simulink model "Motor_Cmd_varY_testHarness"  (Simulink 8.0)
settings: Solver=FixedStepDiscrete  StartTime=0.0  StopTime=10  RelTol=1e-3
PreLoadFcn:
  | Motor_Cmd_varY_selfinit
undefined symbols (not defined in the file): sigbuilder_block
settings Model: SldvGeneratedHarnessModel=TestUnitModel=Motor_Cmd_varY|  Creator=fguerin  LastModifiedBy=klindqvi  RecordCoverage=on  CovMetricSettings=dcoe  CovHTMLOptions=-aTS=1 -bRG=1 -bTC=0 -hTR=0 -nFC=0 -scm=1 -bcm=1 -xEv=0  CovCumulativeReport=on  CovReportOnPause=off  CovModelRefEnable=off  CovExternalEMLEnable=on
settings DataIOCC: ExternalInput=SIM_LockDoorRequest  LimitDataPoints=off  SignalLoggingSaveFormat=ModelDataLogs  SaveOutput=off  DSMLogging=off  SaveTime=off  SignalLoggingName=logsOut
settings OptimizationCC: InlineParams=on  InlineInvariantSignals=on  EnhancedBackFolding=on  ZeroExternalMemoryAtStartup=off  ZeroInternalMemoryAtStartup=off  EfficientFloat2IntCast=on  OptimizeModelRefInitCode=on  LifeSpan=1
settings DebuggingCC: SignalInfNanChecking=error  SignalRangeChecking=error  ReadBeforeWriteMsg=EnableAllAsError  WriteAfterWriteMsg=EnableAllAsError  WriteAfterReadMsg=EnableAllAsError  AlgebraicLoopMsg=error  ArtificialAlgebraicLoopMsg=error  SaveWithDisabledLinksMsg=error  SaveWithParameterizedLinksMsg=error  CheckExecutionContextPreStartOutputMsg=on  CheckExecutionContextRuntimeOutputMsg=on  BlockPriorityViolationMsg=error  SolverPrmCheckMsg=error  MultiTaskCondExecSysMsg=warning  MultiTaskRateTransMsg=warning  CheckMatrixSingularityMsg=error  IntegerOverflowMsg=error  ParameterUnderflowMsg=error  ParameterPrecisionLossMsg=error  ParameterTunabilityLossMsg=error  UnderSpecifiedDataTypeMsg=warning  UnnecessaryDatatypeConvMsg=warning  VectorMatrixConversionMsg=error  FcnCallInpInsideContextMsg=EnableAllAsWarning  SFcnCompatibilityMsg=error  BusObjectLabelMismatch=error  RootOutportRequireBusObject=error  AssertControl=DisableAll  ModelReferenceIOMsg=error  ModelReferenceIOMismatchMessage=error  ModelReferenceCSMismatchMessage=warning  UnknownTsInhSupMsg=error  ModelReferenceDataLoggingMessage=error  StrictBusMsg=ErrorOnBusTreatedAsVector
settings HardwareCC: ProdLargestAtomicInteger=Long  ProdLargestAtomicFloat=Double  ProdIntDivRoundTo=Zero  ProdEndianess=BigEndian  ProdHWDeviceType=Freescale->MPC5500
settings ModelReferenceCC: ModelReferenceNumInstancesAllowed=Single
settings SFSimCC: SimParseCustomCode=off
settings RTWCC: SystemTargetFile=ert.tlc  TemplateMakefile=ert_default_tmf  Description=Embedded Coder  GenerateReport=on  RTWVerbose=off  ProcessScript=ert_make_rtw_hook  IncludeHyperlinkInReport=on  LaunchReport=on  PortableWordSizes=on  GenerateTraceInfo=on  GenerateTraceReport=on  GenerateTraceReportSl=on  GenerateTraceReportSf=on  GenerateTraceReportEml=on  GenerateCodeMetricsReport=on
settings MATStruct: className=coder.coverage.Bullseye  argsAllComponents=[]  excludedModels=[]  includeReferencedModels=off  includeTopModel=on  enabled=on
settings CodeAppCC: ForceParamTrailComments=on  IgnoreCustomStorageClasses=off  IgnoreTestpoints=on  MangleLength=4  InlinedPrmAccess=Macros  ReqsInCode=on
settings ERTTargetCC: CodeReplacementLibrary=ANSI_C  MultiwordLength=2048  GenerateSampleERTMain=on  SupportAbsoluteTime=off  SupportNonFinite=off  SupportComplex=off  InlinedParameterPlacement=NonHierarchical  ERTCustomFileTemplate=example_file_process.tlc  ConvertIfToSwitch=off  SuppressUnreachableDefaultCases=off
settings ConfigComp: Description=Design Verifier Custom Configuration Component  DVMaxProcessTime=600  DVDisplayUnsatisfiableObjectives=on  DVAutomaticStubbing=off  DVOutputDir=C:\Work\Data\Pilots\P_PSA_ECoder_BenchMark_LaGarenne\source9b\deliverable\trunk\demos\VnV_example\Projects\ADL_Project/Simulink_Test_Generation/ADL_Sim  DVModelCoverageObjectives=MCDC  DVTestSuiteOptimization=CombinedObjectives  DVDataFileName=./Tests/$ModelName$_sldvdata  DVSaveHarnessModel=on  DVHarnessModelFileName=./Tests/$ModelName$_testHarness  DVModelReferenceHarness=on  DVSaveReport=on  DVReportFileName=ADL_Sim_SLDV.html

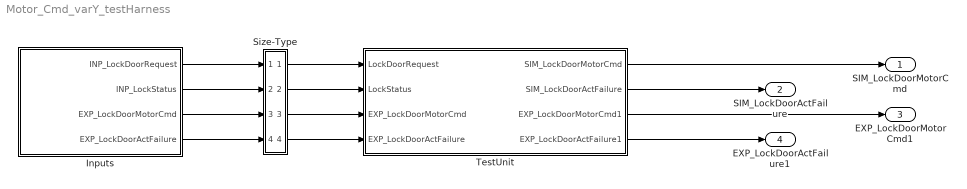
== system Motor_Cmd_varY_testHarness ==
  Inputs : Subsystem  Tag=STV Subsys  RequirementInfo={'other' '..\..\..\..\requirements\doorlockingsystem_swr.doc' '@Simulink_requirement_item_3' 'true' 'REQ301 – A door lock failure should be reported if the door lock has not responded to command in 2 seconds.' '' } %GIDa_ed3108d7_bd27_4d13_a0b7_ca84d234bb27  LoadFcn=sigbuilder_block('load');  StartFcn=sigbuilder_block('start');  StopFcn=sigbuilder_block('stop');  ClipboardFcn=sigbuilder_block('clipboard');  SystemSampleTime=1  mask(Sigbuilder block){}
      mask init:
      | if ~strcmp(get_param(bdroot(gcb),'SimulationStatus'),'stopped'),tuvar = sigbuilder_block('maskInit'); end
      settings: CopyFcn=sigbuilder_block('copy');  DeleteFcn=sigbuilder_block('delete');  ModelCloseFcn=sigbuilder_block('modelClose');  PreSaveFcn=sigbuilder_block('preSave');  PauseFcn=sigbuilder_block('pause')  ContinueFcn=sigbuilder_block('continue')  NameChangeFcn=sigbuilder_block('namechange');  OpenFcn=sigbuilder_block('open',[55.5 107.25 519.75 399.75 ]);  CloseFcn=sigbuilder_block('close');
      mask Display: plot(0, 0, 100, 100,[2, 2, 32, 32, 2], [68, 8, 8, 68, 68],[32, 2], [38, 38], [32, 19, 2],[53, 60, 44], [32, 17, 17, 2],[16, 16, 31, 31]);txt = getActiveGroup(gcbh);text(2, 100, txt,'verticalAlignment', 'top');
  Size-Type : Subsystem
  TestUnit : Subsystem
  SIM_LockDoorMotorCmd : Outport  OutDataTypeStr=uint8  PortDimensions=1
  SIM_LockDoorActFailure : Outport  Port=2  OutDataTypeStr=boolean
  EXP_LockDoorMotorCmd1 : Outport  Port=3  PortDimensions=1
  EXP_LockDoorActFailure1 : Outport  Port=4
  wires:
  Size-Type/1(Out1) -> TestUnit/1(LockDoorRequest)
  Size-Type/2(Out2) -> TestUnit/2(LockStatus)
  Size-Type/3(Out3) -> TestUnit/3(EXP_LockDoorMotorCmd)
  Size-Type/4(Out4) -> TestUnit/4(EXP_LockDoorActFailure)
  TestUnit/1(SIM_LockDoorMotorCmd) -> SIM_LockDoorMotorCmd/1
  TestUnit/2(SIM_LockDoorActFailure) -> SIM_LockDoorActFailure/1
  TestUnit/3(EXP_LockDoorMotorCmd1) -> EXP_LockDoorMotorCmd1/1
  TestUnit/4(EXP_LockDoorActFailure1) -> EXP_LockDoorActFailure1/1
  Inputs/1(INP_LockDoorRequest) -> Size-Type/1(In1)
  Inputs/2(INP_LockStatus) -> Size-Type/2(In2)
  Inputs/3(EXP_LockDoorMotorCmd) -> Size-Type/3(In3)
  Inputs/4(EXP_LockDoorActFailure) -> Size-Type/4(In4)

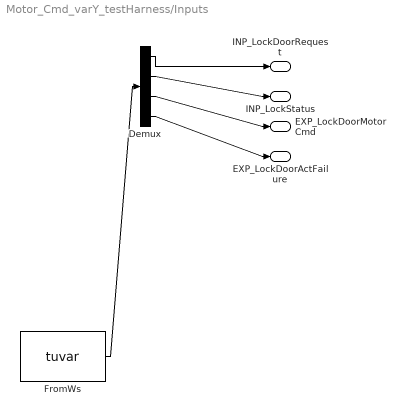
== system Motor_Cmd_varY_testHarness/Inputs ==
  Demux : Demux  Tag=STV Demux
  FromWs : FromWorkspace  Tag=STV FromWs  VariableName=tuvar  SampleTime=0  SigBuilderData=DataTag0  VnvData=DataTag1
      SigBuilderData=|
      | dataSet(1).timeRange = [0 10]
      | dataSet(1).name = 'Test1'
      | dataSet(2).timeRange = [0 10]
      | dataSet(2).name = 'Test2'
      | dataSet(3).timeRange = [0 10]
      | dataSet(3).name = 'Test3'
      | sbobj.Name = 'Signal Builder'
      | sbobj.Groups(1).Name = 'Test1'
      | sbobj.Groups(1).Signals(1).Name = 'INP_LockDoorRequest'
      | sbobj.Groups(1).Signals(1).XData = [0 10]
      | sbobj.Groups(1).Signals(1).YData = [0 0]
      | sbobj.Groups(1).Signals(2).Name = 'INP_LockStatus'
      | sbobj.Groups(1).Signals(2).XData = [0 10]
      | sbobj.Groups(1).Signals(2).YData = [0 0]
      | sbobj.Groups(1).Signals(3).Name = 'EXP_LockDoorMotorCmd'
      | sbobj.Groups(1).Signals(3).XData = [0 10]
      | sbobj.Groups(1).Signals(3).YData = [0 0]
      | sbobj.Groups(1).Signals(4).Name = 'EXP_LockDoorActFailure'
      | sbobj.Groups(1).Signals(4).XData = [0 10]
      | sbobj.Groups(1).Signals(4).YData = [0 0]
      | sbobj.Groups(2).Name = 'Test2'
      | sbobj.Groups(2).Signals(1).Name = 'INP_LockDoorRequest'
      | sbobj.Groups(2).Signals(1).XData = [0 1 1 2 10]
      | sbobj.Groups(2).Signals(1).YData = [0 0 1 1 1]
      | sbobj.Groups(2).Signals(2).Name = 'INP_LockStatus'
      | sbobj.Groups(2).Signals(2).XData = [0 1 1 2 2 10]
      | sbobj.Groups(2).Signals(2).YData = [0 0 0 0 1 1]
      | sbobj.Groups(2).Signals(3).Name = 'EXP_LockDoorMotorCmd'
      | sbobj.Groups(2).Signals(3).XData = [0 1 1 2 2 10]
      | sbobj.Groups(2).Signals(3).YData = [0 0 40 40 40 40]
      | sbobj.Groups(2).Signals(4).Name = 'EXP_LockDoorActFailure'
      | sbobj.Groups(2).Signals(4).XData = [0 1 1 2 2 10]
      | sbobj.Groups(2).Signals(4).YData = [0 0 0 0 0 0]
      | sbobj.Groups(3).Name = 'Test3'
      | sbobj.Groups(3).Signals(1).Name = 'INP_LockDoorRequest'
      | sbobj.Groups(3).Signals(1).XData = [0 1 1 2 10]
      | sbobj.Groups(3).Signals(1).YData = [0 0 1 1 1]
      | sbobj.Groups(3).Signals(2).Name = 'INP_LockStatus'
      | sbobj.Groups(3).Signals(2).XData = [0 1 2 10]
      | sbobj.Groups(3).Signals(2).YData = [0 0 0 0]
      | sbobj.Groups(3).Signals(3).Name = 'EXP_LockDoorMotorCmd'
      | sbobj.Groups(3).Signals(3).XData = [0 1 1 2 10]
      | sbobj.Groups(3).Signals(3).YData = [0 0 40 40 40]
      | sbobj.Groups(3).Signals(4).Name = 'EXP_LockDoorActFailure'
      | sbobj.Groups(3).Signals(4).XData = [0 1 2 3 3 10]
      | sbobj.Groups(3).Signals(4).YData = [0 0 0 0 1 1]
  INP_LockDoorRequest : Outport
  INP_LockStatus : Outport  Tag=STV Outport  Port=2
  EXP_LockDoorMotorCmd : Outport  Tag=STV Outport  Port=3
  EXP_LockDoorActFailure : Outport  Tag=STV Outport  Port=4
  wires:
  FromWs/1 -> Demux/1
  Demux/1 -> INP_LockDoorRequest/1
  Demux/2 -> INP_LockStatus/1
  Demux/3 -> EXP_LockDoorMotorCmd/1
  Demux/4 -> EXP_LockDoorActFailure/1

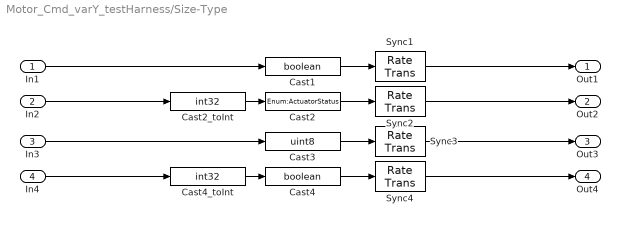
== system Motor_Cmd_varY_testHarness/Size-Type ==
  In1 : Inport
  In2 : Inport  Port=2
  In3 : Inport  Port=3
  In4 : Inport  Port=4
  Cast1 : DataTypeConversion  OutDataTypeStr=boolean  SaturateOnIntegerOverflow=on  RndMeth=Zero
  Cast2 : DataTypeConversion  OutDataTypeStr=Enum:ActuatorStatus  SaturateOnIntegerOverflow=on  RndMeth=Zero
  Cast2_toInt : DataTypeConversion  OutDataTypeStr=int32  SaturateOnIntegerOverflow=on  RndMeth=Zero
  Cast3 : DataTypeConversion  OutDataTypeStr=uint8  SaturateOnIntegerOverflow=on  RndMeth=Zero
  Cast4 : DataTypeConversion  OutDataTypeStr=boolean  SaturateOnIntegerOverflow=on  RndMeth=Zero
  Cast4_toInt : DataTypeConversion  OutDataTypeStr=int32  SaturateOnIntegerOverflow=on  RndMeth=Zero
  Sync{1..4} (4 alike) : RateTransition  OutPortSampleTime=0.5
  Out1 : Outport
  Out2 : Outport  Port=2
  Out3 : Outport  Port=3
  Out4 : Outport  Port=4
  wires:
  In1/1 -> Cast1/1
  Cast1/1 -> Sync1/1
  Sync1/1 -> Out1/1
  In2/1 -> Cast2_toInt/1
  Cast2_toInt/1 -> Cast2/1
  Cast2/1 -> Sync2/1
  Sync2/1 -> Out2/1
  In3/1 -> Cast3/1
  Cast3/1 -> Sync3/1
  Sync3/1 -> Out3/1
  In4/1 -> Cast4_toInt/1
  Cast4_toInt/1 -> Cast4/1
  Cast4/1 -> Sync4/1
  Sync4/1 -> Out4/1

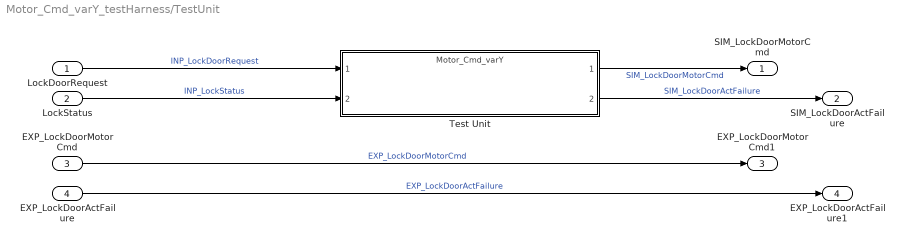
== system Motor_Cmd_varY_testHarness/TestUnit ==
  LockDoorRequest : Inport  OutDataTypeStr=boolean  PortDimensions=1
  LockStatus : Inport  Port=2  OutDataTypeStr=Enum: ActuatorStatus  PortDimensions=1
  EXP_LockDoorMotorCmd : Inport  Port=3  PortDimensions=1
  EXP_LockDoorActFailure : Inport  Port=4  PortDimensions=1
  Test Unit : ModelReference  ModelNameDialog=Motor_Cmd_varY  SimulationMode=Normal  ModelReferenceVersion=1.79  CopyOfModelName=Motor_Cmd_varY  DefaultDataLogging=off
  SIM_LockDoorMotorCmd : Outport  OutDataTypeStr=uint8  PortDimensions=1
  SIM_LockDoorActFailure : Outport  Port=2  OutDataTypeStr=boolean
  EXP_LockDoorMotorCmd1 : Outport  Port=3  PortDimensions=1
  EXP_LockDoorActFailure1 : Outport  Port=4
  wires:
  EXP_LockDoorActFailure/1 -> EXP_LockDoorActFailure1/1  "EXP_LockDoorActFailure"
  EXP_LockDoorMotorCmd/1 -> EXP_LockDoorMotorCmd1/1  "EXP_LockDoorMotorCmd"
  Test Unit/2 -> SIM_LockDoorActFailure/1  "SIM_LockDoorActFailure"
  Test Unit/1 -> SIM_LockDoorMotorCmd/1  "SIM_LockDoorMotorCmd"
  LockStatus/1 -> Test Unit/2  "INP_LockStatus"
  LockDoorRequest/1 -> Test Unit/1  "INP_LockDoorRequest"
